simulink model "ParkingMeterLowLevel"  (R2018b)
settings: Solver=FixedStepAuto  StartTime=0.0  StopTime=Inf  FixedStep=SAMPLING_TIME  RelTol=1e-3
PreLoadFcn:
  | startGUI();
undefined symbols (not defined in the file): BIT_MASK_010_CENTS, BIT_MASK_020_CENTS, BIT_MASK_050_CENTS, BIT_MASK_100_CENTS, BIT_MASK_ADD_LED, BIT_MASK_BOTH_LEDS_NOT, BIT_MASK_COINS_FLAP, BIT_MASK_COINS_FLAP_NOT, BIT_MASK_GREEN_BUTTON, BIT_MASK_MASTER_SWITCH, BIT_MASK_PRINT_TICKET, BIT_MASK_RED_BUTTON, BIT_MASK_RETURN_LED, char2dec, INTEGER_010_CENTS, INTEGER_020_CENTS, INTEGER_050_CENTS, INTEGER_100_CENTS, INTEGER_200_CENTS
libraries: simulink x17, Components x9
CloseFcn:
  | closeGUI();
settings Model: DataDictionary=Parameters.sldd  ModifiedHistory=% Copyright 2018 The MathWorks, Inc.  EnablePacing=on  Creator=sdupertu  LastModifiedBy=sdupertu
settings OptimizationCC: DefaultParameterBehavior=Inlined  EnhancedBackFolding=on  PassReuseOutputArgsAs=Individual arguments  OptimizeBlockOrder=speed  DifferentSizesBufferReuse=on  OptimizationCustomize=off
settings DebuggingCC: UnderspecifiedInitializationDetection=Classic  MergeDetectMultiDrivingBlocksExec=none  ParameterTunabilityLossMsg=error  LibraryContextMissingDiagnostic=none
settings SFSimCC: SimUseLocalCustomCode=off  MATLABDynamicMemAlloc=off
settings RTWCC: SystemTargetFile=ert.tlc  TemplateMakefile=ert_default_tmf  GenerateReport=on  RTWUseLocalCustomCode=off  IncludeHyperlinkInReport=on  LaunchReport=on  GenerateTraceInfo=on  GenerateTraceReport=on  GenerateTraceReportSl=on  GenerateTraceReportSf=on  GenerateTraceReportEml=on  GenerateWebview=on  GenerateCodeMetricsReport=on
settings CodeAppCC: ForceParamTrailComments=on  IgnoreCustomStorageClasses=off  MaxIdLength=61  OperatorAnnotations=on  SimulinkDataObjDesc=on  SFDataObjDesc=on  InsertBlockDesc=on
settings ERTTargetCC: TargetLangStandard=C99 (ISO)  GenerateSampleERTMain=on  InlinedParameterPlacement=NonHierarchical  ERTCustomFileTemplate=example_file_process.tlc

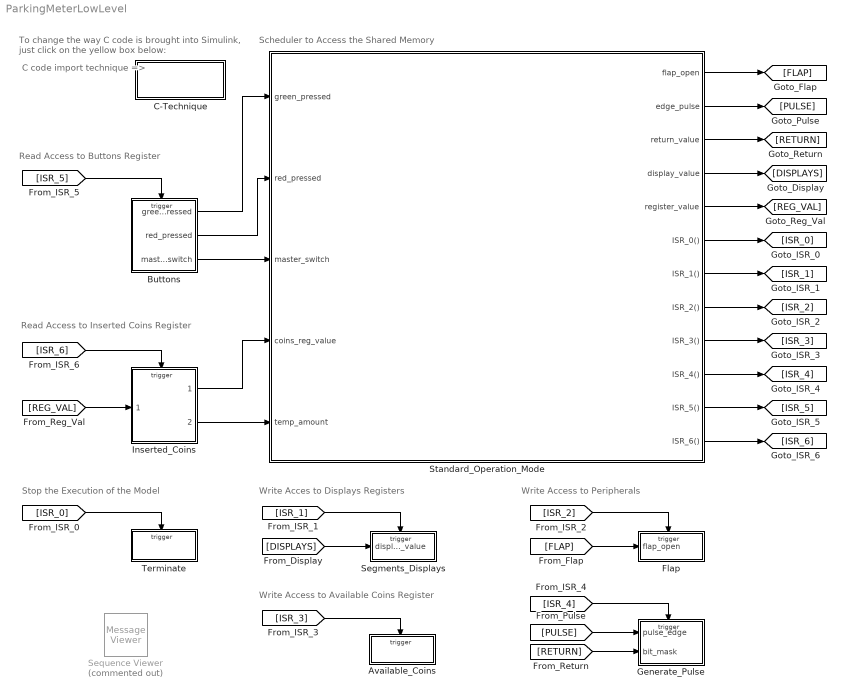
== system ParkingMeterLowLevel ==
  note: To change the way C code is brought into Simulink,
      | just click on the yellow box below:
  note: Stop the Execution of the Model
  note: Scheduler to Access the Shared Memory
  note: Write Access to Available Coins Register
  note: Write Access to Peripherals
  note: Write Acces to Displays Registers
  note: Read Access to Inserted Coins Register
  note: Read Access to Buttons Register
  note: C code import
      | technique =>
  Available_Coins : Subsystem
  Buttons : Subsystem
  C-Technique : Subsystem
      mask Display:
      | % Get the variant that has been selected for the C import
      | load_system('ReadRegister');
      | C_technique = get_param('ReadRegister/read_register','ActiveVariant');
      | if strcmp(C_technique,'SRC')
      |   text_technique = 'C-Caller';
      | elseif strcmp(C_technique,'MEX')
      |   text_technique = 'S-Function';
      | else
      |   text_technique = 'Error';
      | end
      | text(0.5,0.6,['{\bf\fontsize{16}' text_technique '}'],...
      |      'horizontalAlignment','center','texmode','on');
  Flap : Subsystem
  Generate_Pulse : Subsystem
  Inserted_Coins : Subsystem
  Segments_Displays : Subsystem
      settings: PropExecContextOutsideSubsystem=on
  Sequence Viewer : MessageViewer  Commented=on
  Standard_Operation_Mode : Stateflow chart  TreatAsAtomicUnit=on
  Terminate : Subsystem
  wires:
  Standard_Operation_Mode/4(display_value) -> [DISPLAYS]
  Standard_Operation_Mode/7(ISR_1()) -> [ISR_1]
  [ISR_1] -> Segments_Displays/Trigger
  Standard_Operation_Mode/1(flap_open) -> [FLAP]
  Standard_Operation_Mode/8(ISR_2()) -> [ISR_2]
  [ISR_2] -> Flap/Trigger
  Buttons/1(green_pressed) -> Standard_Operation_Mode/1(green_pressed)
  Standard_Operation_Mode/9(ISR_3()) -> [ISR_3]
  [ISR_5] -> Buttons/Trigger
  Standard_Operation_Mode/10(ISR_4()) -> [ISR_4]
  [ISR_3] -> Available_Coins/Trigger
  [DISPLAYS] -> Segments_Displays/1(display_value)
  [FLAP] -> Flap/1(flap_open)
  [ISR_6] -> Inserted_Coins/Trigger
  Standard_Operation_Mode/11(ISR_5()) -> [ISR_5]
  Buttons/2(red_pressed) -> Standard_Operation_Mode/2(red_pressed)
  [REG_VAL] -> Inserted_Coins/1(old_reg_value)
  Inserted_Coins/2(new_amount) -> Standard_Operation_Mode/5(temp_amount)
  Inserted_Coins/1(new_reg_value) -> Standard_Operation_Mode/4(coins_reg_value)
  Standard_Operation_Mode/5(register_value) -> [REG_VAL]
  [PULSE] -> Generate_Pulse/1(pulse_edge)
  Standard_Operation_Mode/2(edge_pulse) -> [PULSE]
  [ISR_4] -> Generate_Pulse/Trigger
  Standard_Operation_Mode/12(ISR_6()) -> [ISR_6]
  Standard_Operation_Mode/3(return_value) -> [RETURN]
  [RETURN] -> Generate_Pulse/2(bit_mask)
  Buttons/3(master_switch) -> Standard_Operation_Mode/3(master_switch)
  Standard_Operation_Mode/6(ISR_0()) -> [ISR_0]
  [ISR_0] -> Terminate/Trigger

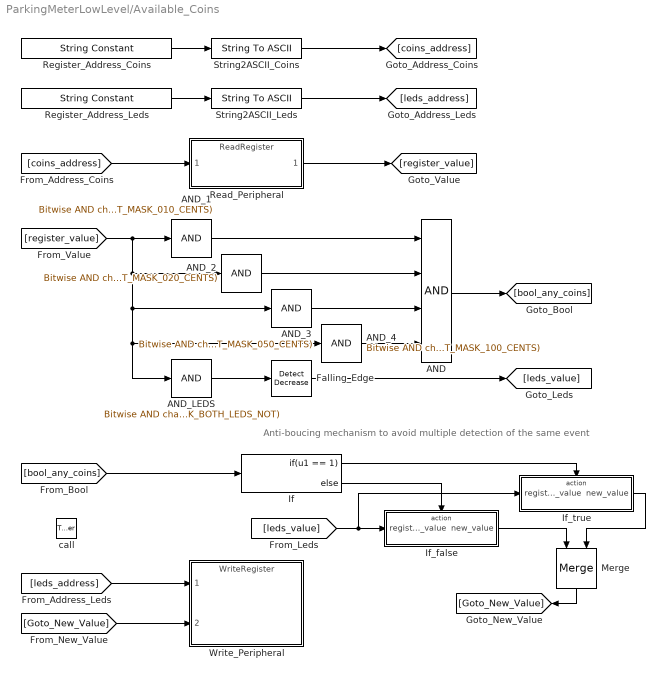
== system ParkingMeterLowLevel/Available_Coins ==
  note: Anti-boucing mechanism to avoid multiple detection of the same event
  call : TriggerPort  TriggerType=function-call  VariantControl=Variant  PortDimensions=1
  AND : Logic  Inputs=4  AllPortsSameDT=off  OutDataTypeStr=boolean
  AND_1 : simulink/Logic and Bit Operations/Bitwise Operator  logicop=AND  UseBitMask=on  BitMask=char2dec(BIT_MASK_010_CENTS)  BitMaskRealWorld=Stored Integer
  AND_2 : simulink/Logic and Bit Operations/Bitwise Operator  logicop=AND  UseBitMask=on  BitMask=char2dec(BIT_MASK_020_CENTS)  BitMaskRealWorld=Stored Integer
  AND_3 : simulink/Logic and Bit Operations/Bitwise Operator  logicop=AND  UseBitMask=on  BitMask=char2dec(BIT_MASK_050_CENTS)  BitMaskRealWorld=Stored Integer
  AND_4 : simulink/Logic and Bit Operations/Bitwise Operator  logicop=AND  UseBitMask=on  BitMask=char2dec(BIT_MASK_100_CENTS)  BitMaskRealWorld=Stored Integer
  AND_LEDS : simulink/Logic and Bit Operations/Bitwise Operator  logicop=AND  UseBitMask=on  BitMask=char2dec(BIT_MASK_BOTH_LEDS_NOT)  BitMaskRealWorld=Stored Integer
  Falling_Edge : simulink/Logic and Bit Operations/Detect Decrease  vinit=0  OutDataTypeStr=uint8
  If : If  IfExpression=u1 == 1
  If_false : Subsystem  TreatAsAtomicUnit=on
  If_true : Subsystem  TreatAsAtomicUnit=on
  Merge : Merge
  Read_Peripheral : ModelReference  ModelNameDialog=ReadRegister  SimulationMode=Normal  ModelReferenceVersion=1.112
  Register_Address_Coins : StringConstant  String=AVAILABLE_COINS_REGISTER
  Register_Address_Leds : StringConstant  String=PERIPHERALS_REGISTER
  String2ASCII_Coins : StringToASCII  MaximumLength=6
  String2ASCII_Leds : StringToASCII  MaximumLength=6
  Write_Peripheral : ModelReference  ModelNameDialog=WriteRegister  SimulationMode=Normal  ModelReferenceVersion=1.129
  wires:
  String2ASCII_Coins/1 -> [coins_address]
  [leds_address] -> Write_Peripheral/1
  Register_Address_Coins/1 -> String2ASCII_Coins/1
  [coins_address] -> Read_Peripheral/1
  Read_Peripheral/1 -> [register_value]
  [Goto_New_Value] -> Write_Peripheral/2
  AND_1/1 -> AND/1
  [register_value] -> AND_LEDS/1, AND_4/1, AND_3/1, AND_2/1, AND_1/1
  AND_3/1 -> AND/3
  AND_2/1 -> AND/2
  AND_4/1 -> AND/4
  AND/1 -> [bool_any_coins]
  If/2 -> If_false/Action
  If_true/1(new_value) -> Merge/2
  [bool_any_coins] -> If/1
  If_false/1(new_value) -> Merge/1
  If/1 -> If_true/Action
  [leds_value] -> If_true/1(register_value), If_false/1(register_value)
  AND_LEDS/1 -> Falling_Edge/1
  Merge/1 -> [Goto_New_Value]
  Register_Address_Leds/1 -> String2ASCII_Leds/1
  String2ASCII_Leds/1 -> [leds_address]
  Falling_Edge/1 -> [leds_value]

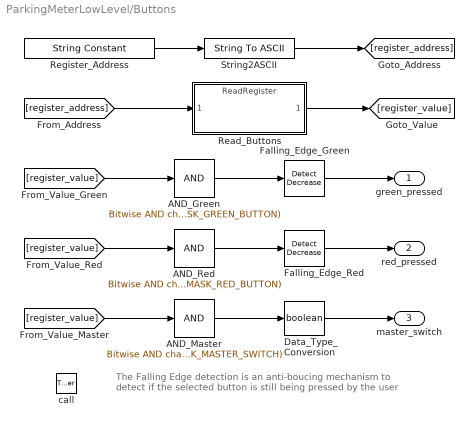
== system ParkingMeterLowLevel/Buttons ==
  note: The Falling Edge detection is an anti-boucing mechanism to
      | detect if the selected button is still being pressed by the user
  call : TriggerPort  TriggerType=function-call  VariantControl=Variant  PortDimensions=1
  AND_Green : simulink/Logic and Bit Operations/Bitwise Operator  logicop=AND  UseBitMask=on  BitMask=char2dec(BIT_MASK_GREEN_BUTTON)  BitMaskRealWorld=Stored Integer
  AND_Master : simulink/Logic and Bit Operations/Bitwise Operator  logicop=AND  UseBitMask=on  BitMask=char2dec(BIT_MASK_MASTER_SWITCH)  BitMaskRealWorld=Stored Integer
  AND_Red : simulink/Logic and Bit Operations/Bitwise Operator  logicop=AND  UseBitMask=on  BitMask=char2dec(BIT_MASK_RED_BUTTON)  BitMaskRealWorld=Stored Integer
  Data_Type_Conversion : DataTypeConversion  OutDataTypeStr=boolean
  Falling_Edge_Green : simulink/Logic and Bit Operations/Detect Decrease  vinit=0  OutDataTypeStr=boolean
  Falling_Edge_Red : simulink/Logic and Bit Operations/Detect Decrease  vinit=0  OutDataTypeStr=boolean
  Read_Buttons : ModelReference  ModelNameDialog=ReadRegister.slx  SimulationMode=Normal  ModelReferenceVersion=1.112
  Register_Address : StringConstant  String=BUTTONS_REGISTER
  String2ASCII : StringToASCII  MaximumLength=6
  green_pressed : Outport
  red_pressed : Outport  Port=2
  master_switch : Outport  Port=3
  wires:
  String2ASCII/1 -> [register_address]
  Register_Address/1 -> String2ASCII/1
  [register_address] -> Read_Buttons/1
  Read_Buttons/1 -> [register_value]
  [register_value] -> AND_Green/1
  AND_Green/1 -> Falling_Edge_Green/1
  Falling_Edge_Green/1 -> green_pressed/1
  AND_Red/1 -> Falling_Edge_Red/1
  Falling_Edge_Red/1 -> red_pressed/1
  [register_value] -> AND_Red/1
  AND_Master/1 -> Data_Type_Conversion/1
  [register_value] -> AND_Master/1
  Data_Type_Conversion/1 -> master_switch/1

== system ParkingMeterLowLevel/C-Technique ==

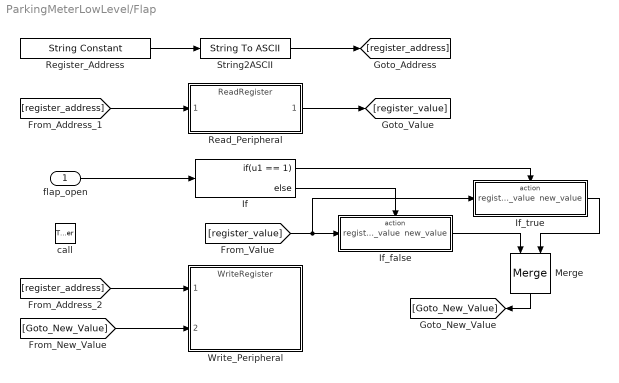
== system ParkingMeterLowLevel/Flap ==
  flap_open : Inport
  call : TriggerPort  TriggerType=function-call  VariantControl=Variant  PortDimensions=1
  If : If  IfExpression=u1 == 1
  If_false : Subsystem  TreatAsAtomicUnit=on
  If_true : Subsystem  TreatAsAtomicUnit=on
  Merge : Merge
  Read_Peripheral : ModelReference  ModelNameDialog=ReadRegister  SimulationMode=Normal  ModelReferenceVersion=1.112
  Register_Address : StringConstant  String=PERIPHERALS_REGISTER
  String2ASCII : StringToASCII  MaximumLength=6
  Write_Peripheral : ModelReference  ModelNameDialog=WriteRegister  SimulationMode=Normal  ModelReferenceVersion=1.129
  wires:
  String2ASCII/1 -> [register_address]
  [register_address] -> Write_Peripheral/1
  Register_Address/1 -> String2ASCII/1
  [register_address] -> Read_Peripheral/1
  Read_Peripheral/1 -> [register_value]
  flap_open/1 -> If/1
  If/1 -> If_true/Action
  [register_value] -> If_true/1(register_value), If_false/1(register_value)
  If/2 -> If_false/Action
  If_false/1(new_value) -> Merge/1
  If_true/1(new_value) -> Merge/2
  Merge/1 -> [Goto_New_Value]
  [Goto_New_Value] -> Write_Peripheral/2

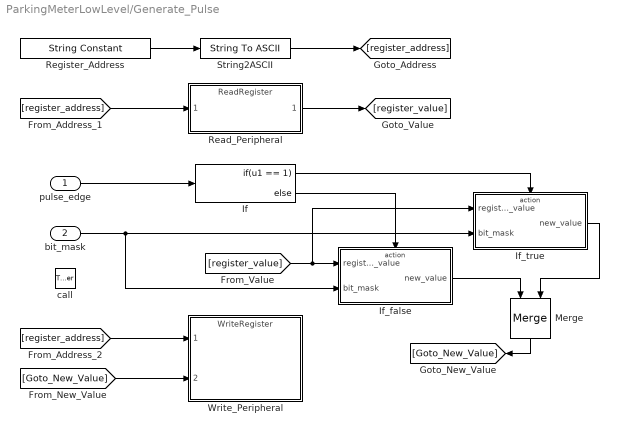
== system ParkingMeterLowLevel/Generate_Pulse ==
  pulse_edge : Inport
  bit_mask : Inport  Port=2
  call : TriggerPort  TriggerType=function-call  VariantControl=Variant  PortDimensions=1
  If : If  IfExpression=u1 == 1
  If_false : Subsystem  TreatAsAtomicUnit=on
  If_true : Subsystem  TreatAsAtomicUnit=on
  Merge : Merge
  Read_Peripheral : ModelReference  ModelNameDialog=ReadRegister  SimulationMode=Normal  ModelReferenceVersion=1.112
  Register_Address : StringConstant  String=PERIPHERALS_REGISTER
  String2ASCII : StringToASCII  MaximumLength=6
  Write_Peripheral : ModelReference  ModelNameDialog=WriteRegister  SimulationMode=Normal  ModelReferenceVersion=1.129
  wires:
  String2ASCII/1 -> [register_address]
  [register_address] -> Write_Peripheral/1
  Register_Address/1 -> String2ASCII/1
  [register_address] -> Read_Peripheral/1
  Read_Peripheral/1 -> [register_value]
  [Goto_New_Value] -> Write_Peripheral/2
  Merge/1 -> [Goto_New_Value]
  If_true/1(new_value) -> Merge/2
  If/2 -> If_false/Action
  [register_value] -> If_true/1(register_value), If_false/1(register_value)
  bit_mask/1 -> If_true/2(bit_mask), If_false/2(bit_mask)
  If_false/1(new_value) -> Merge/1
  pulse_edge/1 -> If/1
  If/1 -> If_true/Action

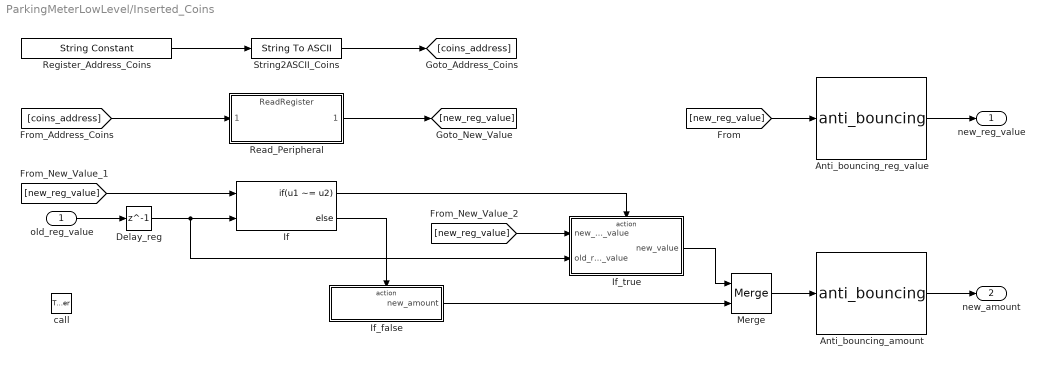
== system ParkingMeterLowLevel/Inserted_Coins ==
  old_reg_value : Inport
  call : TriggerPort  TriggerType=function-call  VariantControl=Variant  PortDimensions=1
  Anti_bouncing_amount : Components/anti_bouncing  SystemSampleTime=-1
  Anti_bouncing_reg_value : Components/anti_bouncing  SystemSampleTime=-1
  Delay_reg : Delay  DelayLength=1  InitialCondition=0
  If : If  NumInputs=2  IfExpression=u1 ~= u2
  If_false : Subsystem  TreatAsAtomicUnit=on
  If_true : Subsystem  TreatAsAtomicUnit=on
  Merge : Merge
  Read_Peripheral : ModelReference  ModelNameDialog=ReadRegister  SimulationMode=Normal  ModelReferenceVersion=1.112
  Register_Address_Coins : StringConstant  String=INSERTED_COINS_REGISTER
  String2ASCII_Coins : StringToASCII  MaximumLength=6
  new_reg_value : Outport
  new_amount : Outport  Port=2
  wires:
  String2ASCII_Coins/1 -> [coins_address]
  Register_Address_Coins/1 -> String2ASCII_Coins/1
  [coins_address] -> Read_Peripheral/1
  Read_Peripheral/1 -> [new_reg_value]
  If/2 -> If_false/Action
  If_true/1(new_value) -> Merge/1
  [new_reg_value] -> If/1
  If_false/1(new_amount) -> Merge/2
  If/1 -> If_true/Action
  [new_reg_value] -> If_true/1(new_reg_value)
  old_reg_value/1 -> Delay_reg/1
  Delay_reg/1 -> If_true/2(old_reg_value), If/2
  Merge/1 -> Anti_bouncing_amount/1
  Anti_bouncing_amount/1 -> new_amount/1
  [new_reg_value] -> Anti_bouncing_reg_value/1
  Anti_bouncing_reg_value/1 -> new_reg_value/1

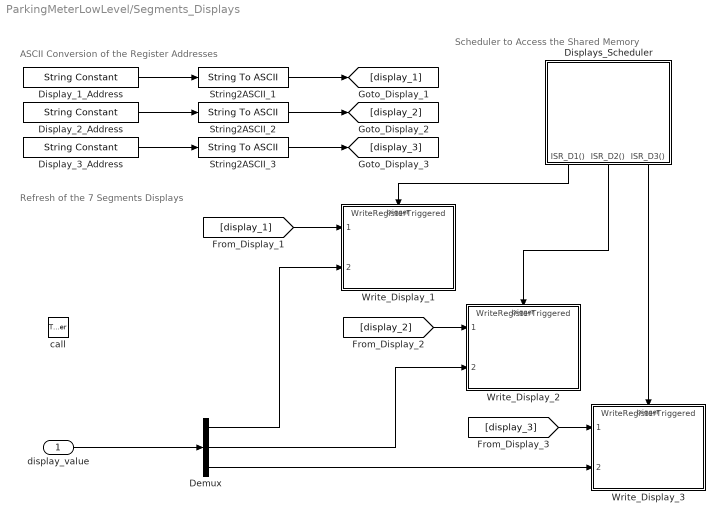
== system ParkingMeterLowLevel/Segments_Displays ==
  note: Scheduler to Access the Shared Memory
  note: Refresh of the 7 Segments Displays
  note: ASCII Conversion of the Register Addresses
  display_value : Inport
  call : TriggerPort  TriggerType=function-call  VariantControl=Variant  SampleTime=-1  PortDimensions=1
  Demux : Demux  Outputs=3
  Display_1_Address : StringConstant  String=DISPLAY_REGISTER_1
  Display_2_Address : StringConstant  String=DISPLAY_REGISTER_2
  Display_3_Address : StringConstant  String=DISPLAY_REGISTER_3
  Displays_Scheduler : Stateflow chart  TreatAsAtomicUnit=on
  String2ASCII_1 : StringToASCII  MaximumLength=6
  String2ASCII_2 : StringToASCII  MaximumLength=6
  String2ASCII_3 : StringToASCII  MaximumLength=6
  Write_Display_1 : ModelReference  ModelNameDialog=WriteRegisterTriggered  SimulationMode=Normal  ModelReferenceVersion=1.124  TriggerPortName=trigger  TriggerPortTriggerType=function-call  TriggerPortStatesWhenEnabling=held
  Write_Display_2 : ModelReference  ModelNameDialog=WriteRegisterTriggered  SimulationMode=Normal  ModelReferenceVersion=1.124  TriggerPortName=trigger  TriggerPortTriggerType=function-call  TriggerPortStatesWhenEnabling=held
  Write_Display_3 : ModelReference  ModelNameDialog=WriteRegisterTriggered  SimulationMode=Normal  ModelReferenceVersion=1.124  TriggerPortName=trigger  TriggerPortTriggerType=function-call  TriggerPortStatesWhenEnabling=held
  wires:
  Demux/2 -> Write_Display_2/2
  Demux/3 -> Write_Display_3/2
  Demux/1 -> Write_Display_1/2
  display_value/1 -> Demux/1
  Displays_Scheduler/1(ISR_D1()) -> Write_Display_1/Trigger
  Displays_Scheduler/2(ISR_D2()) -> Write_Display_2/Trigger
  Displays_Scheduler/3(ISR_D3()) -> Write_Display_3/Trigger
  Display_2_Address/1 -> String2ASCII_2/1
  Display_1_Address/1 -> String2ASCII_1/1
  Display_3_Address/1 -> String2ASCII_3/1
  String2ASCII_1/1 -> [display_1]
  String2ASCII_2/1 -> [display_2]
  String2ASCII_3/1 -> [display_3]
  [display_1] -> Write_Display_1/1
  [display_2] -> Write_Display_2/1
  [display_3] -> Write_Display_3/1

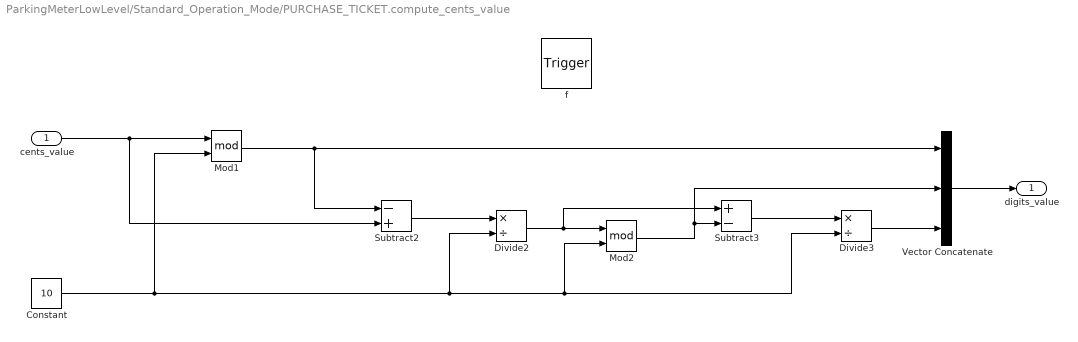
== system ParkingMeterLowLevel/Standard_Operation_Mode/PURCHASE_TICKET.compute_cents_value ==
  cents_value : Inport  OutDataTypeStr=uint8  PortDimensions=[1 1]
  f : TriggerPort  TriggerType=function-call  VariantControl=(inherit)
      settings: CopyFcn=Stateflow.SLINSF.SimulinkMan.removeBlockPreDeleteFcn  PreDeleteFcn=Stateflow.SLINSF.SimulinkMan.unsafePredeleteFcn
  Constant : Constant  Value=10  OutDataTypeStr=uint8
  Divide2 : Product  Inputs=*/
  Divide3 : Product  Inputs=*/
  Mod1 : Math  Operator=mod  SaturateOnIntegerOverflow=on
  Mod2 : Math  Operator=mod  SaturateOnIntegerOverflow=on
  Subtract2 : Sum  Inputs=-+
  Subtract3 : Sum  Inputs=+-
  Vector Concatenate : Concatenate  NumInputs=3
  digits_value : Outport  PortDimensions=[1 3]
  wires:
  cents_value/1 -> Mod1/1, Subtract2/2
  Mod1/1 -> Subtract2/1, Vector Concatenate/1
  Vector Concatenate/1 -> digits_value/1
  Subtract2/1 -> Divide2/1
  Divide2/1 -> Subtract3/1, Mod2/1
  Mod2/1 -> Subtract3/2, Vector Concatenate/2
  Divide3/1 -> Vector Concatenate/3
  Constant/1 -> Mod2/2, Divide3/2, Divide2/2, Mod1/2
  Subtract3/1 -> Divide3/1

== system ParkingMeterLowLevel/Terminate ==
  call : TriggerPort  TriggerType=function-call  VariantControl=Variant  PortDimensions=1
  MATLAB Function : MATLAB Function  TreatAsAtomicUnit=on

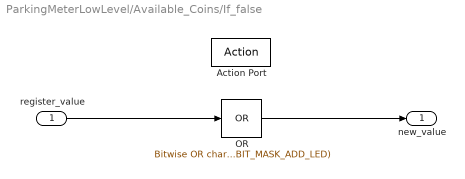
== system ParkingMeterLowLevel/Available_Coins/If_false ==
  register_value : Inport
  Action Port : ActionPort  ActionType=else
  OR : simulink/Logic and Bit Operations/Bitwise Operator  logicop=OR  UseBitMask=on  BitMask=char2dec(BIT_MASK_ADD_LED)  BitMaskRealWorld=Stored Integer
  new_value : Outport
  wires:
  register_value/1 -> OR/1
  OR/1 -> new_value/1

== system ParkingMeterLowLevel/Available_Coins/If_true ==
  register_value : Inport
  Action Port : ActionPort  ActionType=then
  OR : simulink/Logic and Bit Operations/Bitwise Operator  logicop=OR  UseBitMask=on  BitMask=char2dec(BIT_MASK_RETURN_LED)  BitMaskRealWorld=Stored Integer
  new_value : Outport
  wires:
  register_value/1 -> OR/1
  OR/1 -> new_value/1

== system ParkingMeterLowLevel/Flap/If_false ==
  register_value : Inport
  Action Port : ActionPort  ActionType=else
  AND : simulink/Logic and Bit Operations/Bitwise Operator  logicop=AND  UseBitMask=on  BitMask=char2dec(BIT_MASK_COINS_FLAP_NOT)  BitMaskRealWorld=Stored Integer
  new_value : Outport
  wires:
  register_value/1 -> AND/1
  AND/1 -> new_value/1

== system ParkingMeterLowLevel/Flap/If_true ==
  register_value : Inport
  Action Port : ActionPort  ActionType=then
  OR : simulink/Logic and Bit Operations/Bitwise Operator  logicop=OR  UseBitMask=on  BitMask=char2dec(BIT_MASK_COINS_FLAP)  BitMaskRealWorld=Stored Integer
  new_value : Outport
  wires:
  register_value/1 -> OR/1
  OR/1 -> new_value/1

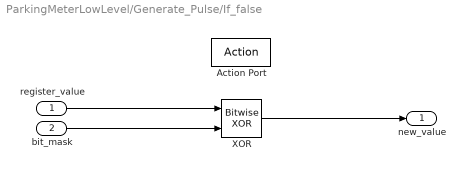
== system ParkingMeterLowLevel/Generate_Pulse/If_false ==
  register_value : Inport
  bit_mask : Inport  Port=2
  Action Port : ActionPort  ActionType=else
  XOR : simulink/Logic and Bit Operations/Bitwise Operator  logicop=XOR  UseBitMask=off  NumInputPorts=2  BitMask=char2dec(BIT_MASK_PRINT_TICKET)  BitMaskRealWorld=Stored Integer
  new_value : Outport
  wires:
  register_value/1 -> XOR/1
  XOR/1 -> new_value/1
  bit_mask/1 -> XOR/2

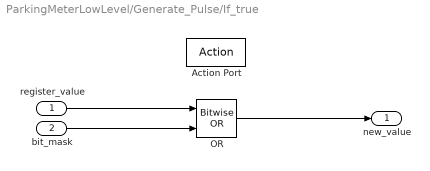
== system ParkingMeterLowLevel/Generate_Pulse/If_true ==
  register_value : Inport
  bit_mask : Inport  Port=2
  Action Port : ActionPort  ActionType=then
  OR : simulink/Logic and Bit Operations/Bitwise Operator  logicop=OR  UseBitMask=off  NumInputPorts=2  BitMask=char2dec(BIT_MASK_PRINT_TICKET)  BitMaskRealWorld=Stored Integer
  new_value : Outport
  wires:
  register_value/1 -> OR/1
  OR/1 -> new_value/1
  bit_mask/1 -> OR/2

== system ParkingMeterLowLevel/Inserted_Coins/If_false ==
  Action Port : ActionPort  ActionType=else
  Constant_0 : Constant  Value=uint8(0)
  new_amount : Outport  InitialOutput=0
  wires:
  Constant_0/1 -> new_amount/1

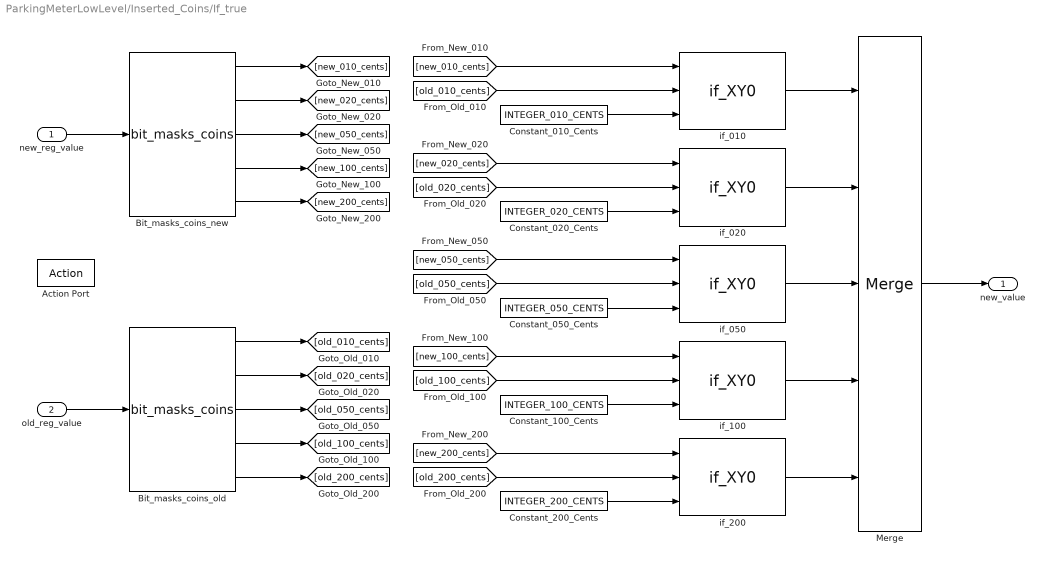
== system ParkingMeterLowLevel/Inserted_Coins/If_true ==
  new_reg_value : Inport
  old_reg_value : Inport  Port=2
  Action Port : ActionPort  ActionType=then
  Bit_masks_coins_new : Components/bit_masks_coins  SystemSampleTime=-1
  Bit_masks_coins_old : Components/bit_masks_coins  SystemSampleTime=-1
  Constant_010_Cents : Constant  Value=INTEGER_010_CENTS
  Constant_020_Cents : Constant  Value=INTEGER_020_CENTS
  Constant_050_Cents : Constant  Value=INTEGER_050_CENTS
  Constant_100_Cents : Constant  Value=INTEGER_100_CENTS
  Constant_200_Cents : Constant  Value=INTEGER_200_CENTS
  Merge : Merge  Inputs=5
  if_010 : Components/if_XY0  SystemSampleTime=-1
  if_020 : Components/if_XY0  SystemSampleTime=-1
  if_050 : Components/if_XY0  SystemSampleTime=-1
  if_100 : Components/if_XY0  SystemSampleTime=-1
  if_200 : Components/if_XY0  SystemSampleTime=-1
  new_value : Outport
  wires:
  new_reg_value/1 -> Bit_masks_coins_new/1
  old_reg_value/1 -> Bit_masks_coins_old/1
  Bit_masks_coins_new/1 -> [new_010_cents]
  Bit_masks_coins_new/2 -> [new_020_cents]
  Bit_masks_coins_new/4 -> [new_100_cents]
  Bit_masks_coins_new/3 -> [new_050_cents]
  Bit_masks_coins_old/1 -> [old_010_cents]
  Bit_masks_coins_old/4 -> [old_100_cents]
  Bit_masks_coins_old/3 -> [old_050_cents]
  Bit_masks_coins_old/2 -> [old_020_cents]
  [new_020_cents] -> if_020/1
  [old_020_cents] -> if_020/2
  [new_050_cents] -> if_050/1
  [old_050_cents] -> if_050/2
  [new_100_cents] -> if_100/1
  [old_100_cents] -> if_100/2
  if_050/1 -> Merge/3
  if_020/1 -> Merge/2
  if_100/1 -> Merge/4
  Merge/1 -> new_value/1
  [new_200_cents] -> if_200/1
  if_200/1 -> Merge/5
  [old_200_cents] -> if_200/2
  Bit_masks_coins_old/5 -> [old_200_cents]
  Bit_masks_coins_new/5 -> [new_200_cents]
  [new_010_cents] -> if_010/1
  [old_010_cents] -> if_010/2
  if_010/1 -> Merge/1
  Constant_010_Cents/1 -> if_010/3
  Constant_020_Cents/1 -> if_020/3
  Constant_050_Cents/1 -> if_050/3
  Constant_100_Cents/1 -> if_100/3
  Constant_200_Cents/1 -> if_200/3

== stateflow chart ParkingMeterLowLevel/Segments_Displays/Displays_Scheduler ==
  state Update_DISP1
    entry: % Refresh the status of the first digits display
    send(ISR_D1);
  state Update_DISP2
    entry: % Refresh the status of the second digits display
    send(ISR_D2);
  state Update_DISP3
    entry: % Refresh the status of the third digits display
    send(ISR_D3);
  (default) -> Update_DISP1
  (junction 16) -> Update_DISP1
  (junction 17) -> (junction 16) : [after(2, tick)]
  Update_DISP1 -> Update_DISP2 : [after(2, tick)]
  Update_DISP2 -> Update_DISP3 : [after(2, tick)]
  Update_DISP3 -> (junction 17)
  events: ISR_D1 output FUNCTION_CALL_EVENT; ISR_D2 output FUNCTION_CALL_EVENT; ISR_D3 output FUNCTION_CALL_EVENT

== matlab function ParkingMeterLowLevel/Terminate/MATLAB Function ==
function stopSIM
  %#codegen
  coder.extrinsic('set_param','bdroot');
  if coder.target('Rtw')
  fprintf('The Master Switch of the Parking Meter Interface is switched off.\n');
  fprintf('Therefore the application has stopped and it can be closed.\n');
  % Include the header file containing the needed function declaration
  coder.cinclude('stdlib.h');
  % Stop the main standalone executable properly
  coder.ceval('exit',int32(0));
  else
  % Stop the simulation of the main model properly
  set_param(bdroot, 'SimulationCommand', 'stop');
  end
end

== stateflow chart ParkingMeterLowLevel/Standard_Operation_Mode ==
  state INITIALIZATION
    during: % Reset of the parking meter status
    display_value = uint8(double(SEGMENTS_DIGIT_M)*ones(1,NB_DISP));
    flap_open = logical(0);
    send(ISR_1); % Initial state of the 7 segments displays
    send(ISR_2); % Close the coin's flap
  state PURCHASE_CHECK
    entry: % Waiting on a ticket purchase request
    send(ISR_3); % Ignit the checking of the money that can be given back
    send(ISR_5); % Ignit the checking of the green button and master switch
    during:
    send(ISR_3); % Leds: check if the parking meter can give money back
    send(ISR_5); % Check the status of the green button and master switch
  state STOP_EXECUTION
    during: % Stop the model execution
    send(ISR_0); % Trigger the terminate function to stop the execution
  state CHECK_COINS
    entry: % Update of the button value state once it has been pressed
    send(ISR_5); % Status of the green button must be equal to zero
    during:
    display_value = [SEGMENTS_DIGIT_0, SEGMENTS_DIGIT_2, ...
    SEGMENTS_DIGIT_1+SEGMENTS_DIGIT_P];
    flap_open = logical(1);
    % Send interrupts
    send(ISR_1); % Display the cost of a parking ticket
    send(ISR_2); % Open the coin's flap
  state PURCHASE_TICKET
    % Waiting for the full paiment or the cancellation of the ticket
    state digits_value = compute_cents_value(cents_value) [function]
    state INITIALIZATION
      during: % Reset local variables and pause the process
      inserted_amount = uint16(0);
      amount_to_return = uint8(0);
      register_value = uint8(0);
      remaining_amount = uint8(zeros(1,3));
    state CANCEL_CHECK
      during: % Check if the purchase is being cancelled
      send(ISR_5); % Check status of the red button
    state CANCEL_PURCHASE
      during: % Ticket's purchase process cancelled
      amount_to_return = uint8(inserted_amount);
    state COIN_CHECK
      during: % Update the amount to pay if a coin has been inserted
      send(ISR_6); % Check current inserted coin
      inserted_amount = inserted_amount + uint16(temp_amount);
    state COINS_RISING_EDGE
      entry: % Update the amount to pay if a coin has been inserted
      [amount_to_return, return_value] = ...
      return_coins_value(int32(amount_to_return));
      exit:
      edge_pulse = logical(1);
      send(ISR_4); % Rising Edge of the pulse for the coins to give back
    state UPDATE_AMOUNT
      during: % Update the amount to pay if a coin has been inserted
      register_value = coins_reg_value;
      remaining_amount = ...
      compute_cents_value(uint8(TICKET_FEE-inserted_amount));
      display_value = display_digits(remaining_amount);
      display_value(end) = display_value(end)+SEGMENTS_DIGIT_P;
      send(ISR_1); % Update the remaining cents amount to pay
    state COINS_FALLING_EDGE
      exit: % Generate peripherals pulse
      edge_pulse = logical(0);
      send(ISR_4); % Falling Edge of the pulse for the coins to give back
    state COINS_REMAINING
      during: % Remaining coins to give back
    state TICKET_PAID
      during: % Printing of the parking ticket
      display_value = [SEGMENTS_DIGIT_0, SEGMENTS_DIGIT_0, ...
      SEGMENTS_DIGIT_0+SEGMENTS_DIGIT_P];
      send(ISR_1); % Total ticket amount paid
    state RECEIPT_RISING_EDGE
      exit: % Generate peripherals pulse
      edge_pulse = logical(1);
      return_value = INT_MASK_PRINT_TICKET;
      send(ISR_4); % Rising Edge of the pulse for the receipt
    state RECEIPT_FALLING_EDGE
      exit: % Generate peripherals pulse
      edge_pulse = logical(0);
      send(ISR_4); % Falling Edge of the pulse for the receipt
    state GIVE_BACK_CHANGE
      entry: % Give back coin's change
      amount_to_return = uint8(inserted_amount-TICKET_FEE);
    (default) -> PURCHASE_TICKET.INITIALIZATION
    PURCHASE_TICKET.INITIALIZATION -> CANCEL_CHECK : [after(REFRESHING_TIME, sec)]
    CANCEL_CHECK -> CANCEL_PURCHASE [order 1] : [red_pressed == true]
    (junction 96) -> CANCEL_CHECK
    (junction 97) -> (junction 96) : [after(REFRESHING_TIME, sec)]
    CANCEL_PURCHASE -> COINS_RISING_EDGE : [after(REFRESHING_TIME, sec)]
    COIN_CHECK -> CANCEL_CHECK [order 2] : [after(REFRESHING_TIME, sec)]
    CANCEL_CHECK -> COIN_CHECK [order 2] : [after(REFRESHING_TIME, sec)]
    (junction 153) -> COINS_RISING_EDGE
    COIN_CHECK -> UPDATE_AMOUNT [order 1] : [coins_reg_value ~= register_value]
    (junction 154) -> (junction 153) : [amount_to_return > 0]
    COINS_RISING_EDGE -> COINS_FALLING_EDGE : [after(PULSE_DURATION, sec)]
    UPDATE_AMOUNT -> (junction 97) [order 1]
    COINS_FALLING_EDGE -> COINS_REMAINING : [after(PULSE_DURATION, sec)]
    UPDATE_AMOUNT -> TICKET_PAID [order 2] : [inserted_amount >= TICKET_FEE]
    COINS_REMAINING -> (junction 154) [order 1]
    GIVE_BACK_CHANGE -> COINS_REMAINING : [true]
    TICKET_PAID -> RECEIPT_RISING_EDGE : [after(REFRESHING_TIME, sec)]
    RECEIPT_RISING_EDGE -> RECEIPT_FALLING_EDGE : [after(PULSE_DURATION, sec)]
    RECEIPT_FALLING_EDGE -> GIVE_BACK_CHANGE : [after(PULSE_DURATION, sec)]
  (default) -> INITIALIZATION
  (junction 59) -> INITIALIZATION
  (junction 58) -> (junction 59)
  INITIALIZATION -> PURCHASE_CHECK : [after(REFRESHING_TIME, sec)]
  PURCHASE_CHECK -> (junction 164) [order 1] : [master_switch == false]
  (junction 164) -> STOP_EXECUTION
  PURCHASE_CHECK -> CHECK_COINS [order 2] : [green_pressed == true]
  CHECK_COINS -> PURCHASE_TICKET : [after(REFRESHING_TIME, sec)]
  COINS_REMAINING -> (junction 58) [order 2]
  data: cents_value function_input uint8 size=[1 1]; digits_value function_output size=[1 3]; new_reg_value function_output; digit_value function_input; amount_back function_output; new_reg_value function_output; amount function_input; flap_open output boolean =false; edge_pulse output boolean =false; return_value output; display_value output uint8 size=[1 3]; SEGMENTS_DIGIT_M data_store_memory; SEGMENTS_DIGIT_1 data_store_memory; green_pressed input boolean size=[1 1]; SEGMENTS_DIGIT_0 data_store_memory; SEGMENTS_DIGIT_2 data_store_memory; SEGMENTS_DIGIT_P data_store_memory; REFRESHING_TIME data_store_memory; TICKET_FEE data_store_memory; red_pressed input boolean size=[1 1]; master_switch input boolean size=[1 1]; coins_reg_value input; NB_DISP constant uint8 =uint8(3); temp_amount input; remaining_amount local; SEGMENTS_DIGIT_3 data_store_memory; SEGMENTS_DIGIT_4 data_store_memory; SEGMENTS_DIGIT_5 data_store_memory; SEGMENTS_DIGIT_6 data_store_memory; SEGMENTS_DIGIT_7 data_store_memory; SEGMENTS_DIGIT_8 data_store_memory; SEGMENTS_DIGIT_9 data_store_memory; SEGMENTS_DIGIT_E data_store_memory; INT_CASE_ENTRY_0 data_store_memory; INT_CASE_ENTRY_1 data_store_memory; INT_CASE_ENTRY_2 data_store_memory; INT_CASE_ENTRY_3 data_store_memory; INT_CASE_ENTRY_4 data_store_memory; INT_CASE_ENTRY_5 data_store_memory; INT_CASE_ENTRY_6 data_store_memory; INT_CASE_ENTRY_7 data_store_memory; INT_CASE_ENTRY_8 data_store_memory; INT_CASE_ENTRY_9 data_store_memory; INT_CASE_ENTRY_M data_store_memory; inserted_amount local uint16; register_value output; PULSE_DURATION data_store_memory; amount_to_return local; INT_VAL_010_CENTS data_store_memory; INT_VAL_020_CENTS data_store_memory; INT_VAL_050_CENTS data_store_memory; INT_VAL_100_CENTS data_store_memory; INT_MASK_100_CENTS data_store_memory; INT_MASK_010_CENTS data_store_memory; INT_MASK_020_CENTS data_store_memory; INT_MASK_050_CENTS data_store_memory; INT_MASK_PRINT_TICKET data_store_memory
  events: ISR_0 output FUNCTION_CALL_EVENT; ISR_1 output FUNCTION_CALL_EVENT; ISR_2 output FUNCTION_CALL_EVENT; ISR_3 output FUNCTION_CALL_EVENT; ISR_4 output FUNCTION_CALL_EVENT; ISR_5 output FUNCTION_CALL_EVENT; ISR_6 output FUNCTION_CALL_EVENT
  function new_reg_value = display_digits(digit_value):
    | function new_reg_value = display_digits(digit_value)
    | %%%%%%%%%%%%%%%%%%%%%%%%%%%%%%%%%%%%%%%%%%%%%%%%%%%%%%%%%%%%%%%%%%%%%%%%%%%%%%%%
    | % Function display_digits()
    | % Goal  : Update the 7 segments displays with new digits values
    | % IN    : - digit_value: base 10 value to display on the 7 segments displays
    | % IN/OUT: -
    | % OUT   : - new_reg_value: array of integers representing the updated amount of
    | %           inserted coins
    | %%%%%%%%%%%%%%%%%%%%%%%%%%%%%%%%%%%%%%%%%%%%%%%%%%%%%%%%%%%%%%%%%%%%%%%%%%%%%%%%
    | %#codegen
    |   new_reg_value = uint8(double(SEGMENTS_DIGIT_E)*ones(1,NB_DISP));
    | 
    |   for i=1:1:NB_DISP
    |     switch (digit_value(i))
    |       case INT_CASE_ENTRY_0
    |         new_reg_value(i) = SEGMENTS_DIGIT_0;
    |       case INT_CASE_ENTRY_1
    |         new_reg_value(i) = SEGMENTS_DIGIT_1;
    |       case INT_CASE_ENTRY_2
    |         new_reg_value(i) = SEGMENTS_DIGIT_2;
    |       case INT_CASE_ENTRY_3
    |         new_reg_value(i) = SEGMENTS_DIGIT_3;
    |       case INT_CASE_ENTRY_4
    |         new_reg_value(i) = SEGMENTS_DIGIT_4;
    |       case INT_CASE_ENTRY_5
    |         new_reg_value(i) = SEGMENTS_DIGIT_5;
    |       case INT_CASE_ENTRY_6
    |         new_reg_value(i) = SEGMENTS_DIGIT_6;
    |       case INT_CASE_ENTRY_7
    |         new_reg_value(i) = SEGMENTS_DIGIT_7;
    |       case INT_CASE_ENTRY_8
    |         new_reg_value(i) = SEGMENTS_DIGIT_8;
    |       case INT_CASE_ENTRY_9
    |         new_reg_value(i) = SEGMENTS_DIGIT_9;
    |       case INT_CASE_ENTRY_M
    |         new_reg_value(i) = SEGMENTS_DIGIT_M;
    |       otherwise
    |         % Incorrect 7 segments encoded value given to the selected HW register
    |         new_reg_value(i) = SEGMENTS_DIGIT_E;
    |     end
    |   end
    | end
  function [amount_back, new_reg_value] = return_coins_value(amount):
    | function [amount_back, new_reg_value] = return_coins_value(amount)
    | %%%%%%%%%%%%%%%%%%%%%%%%%%%%%%%%%%%%%%%%%%%%%%%%%%%%%%%%%%%%%%%%%%%%%%%%%%%%%%%%
    | % Function return_coins_value()
    | % Goal  : 
    | % IN    : - amount: amount corresponding to the coin value to return
    | % IN/OUT: -
    | % OUT   : - new_reg_value: value representing the coin's value to return
    | %%%%%%%%%%%%%%%%%%%%%%%%%%%%%%%%%%%%%%%%%%%%%%%%%%%%%%%%%%%%%%%%%%%%%%%%%%%%%%%%
    | %#codegen
    |   new_reg_value = uint8(0);
    |   amount_back   = uint8(0);
    | 
    |   if (amount - INT_VAL_100_CENTS >= 0)
    |     new_reg_value = INT_MASK_100_CENTS;
    |     amount_back = uint8(amount - INT_VAL_100_CENTS);
    |   elseif (amount - INT_VAL_050_CENTS >= 0)
    |     new_reg_value = INT_MASK_050_CENTS;
    |     amount_back = uint8(amount - INT_VAL_050_CENTS);
    |   elseif (amount - INT_VAL_020_CENTS >= 0)
    |     new_reg_value = INT_MASK_020_CENTS;
    |     amount_back = uint8(amount - INT_VAL_020_CENTS);
    |   elseif (amount - INT_VAL_010_CENTS >= 0)
    |     new_reg_value = INT_MASK_010_CENTS;
    |     amount_back = uint8(amount - INT_VAL_010_CENTS);
    |   end
    | end
